simulink model "fir_ssr"  (R2023a)
settings: Solver=VariableStepAuto  StartTime=0.0  StopTime=5000  RelTol=1e-3
PreLoadFcn:
  | xmcCheckSlxPath(bdroot)
  | SSR4_init
InitFcn:
  | xmcCheckSlxPath(bdroot)
  | SSR4_init;
undefined symbols (not defined in the file): N, None, S, SHIFT_ACC, Taps, vsva2197, xcvc1902
libraries: aieBasic x8, aieUtilities x4, dspsrcs4 x1, simulink x1, vmcUtilities x1, aieDSP x1
settings Model: Creator=oliviert  LastModifiedBy=robg
settings SolverCC: AlgebraicLoopSolver=TrustRegion
settings DebuggingCC: UnconnectedInputMsg=warning  UnconnectedOutputMsg=warning  UnconnectedLineMsg=warning
settings ModelReferenceCC: EnableRefExpFcnMdlSchedulingChecks=on
settings RTWCC: DLArmComputeVersion=19.05

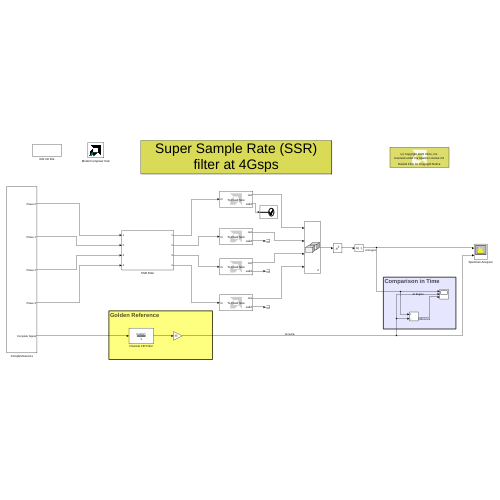
[thumbnail: Simulink's stored preview of the top-level diagram]
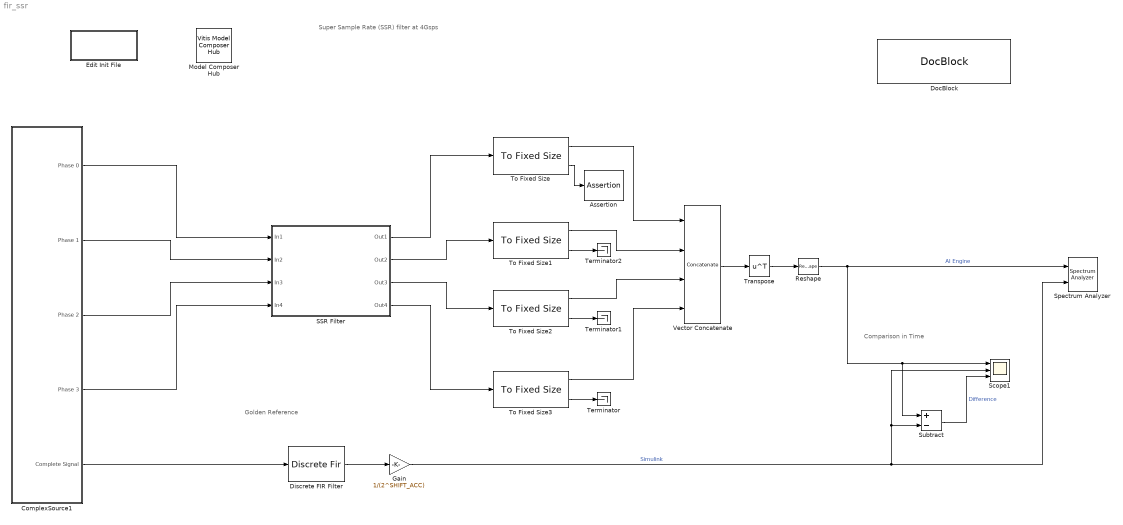
== system fir_ssr ==
  note: Comparison in Time
  note: Golden Reference
  note: Super Sample Rate (SSR) filter at 4Gsps
  Assertion : Assertion
  ComplexSource1 : Subsystem  mask{s=0}
      mask prompts: s "Seed"
  Discrete FIR Filter : DiscreteFir  Coefficients=Taps  InputProcessing=Columns as channels (frame based)
  DocBlock : simulink/Model-Wide Utilities/DocBlock  DocumentType=Text  mask(DocBlock){}
      content=|
      | ///////////////////////////////////////////////////////////////////////////
      | // Copyright 2020 Xilinx
      | //
      | // Licensed under the Apache License, Version 2.0 (the "License");
      | // you may not use this file except in compliance with the License.
      | // You may obtain a copy of the License at
      | //
      | // http://www.apache.org/licenses/LICENSE-2.0
      | //
      | // Unless required by applicable law or agreed to in writing, software
      | // distributed under the License is distributed on an "AS IS" BASIS,
      | // WITHOUT WARRANTIES OR CONDITIONS OF ANY KIND, either express or implied.
      | // See the License for the specific language governing permissions and
      | // limitations under the License.
      | ///////////////////////////////////////////////////////////////////////////
      mask Display:
      | xmcDrawBlockIcon();
      | disp(['{\fontsize{10pt}(c) Copyright 2022' ' Xilinx, Inc.}\newline \newline '],'texmode','on');
      | disp('{\fontsize{10pt}Licensed under the Apache License 2.0}','texmode','on');
      | disp('\newline \newline \newline{\fontsize{10pt}Double Click for Copyright Notice}','texmode','on');
  Edit Init File : Subsystem
      settings: OpenFcn=edit('SSR4_init.m');
  Gain : Gain  Gain=1/(2^SHIFT_ACC)
  Model Composer Hub : vmcUtilities/Vitis Model Composer Hub  Tag=genX  CodeGeneration=off  SubsystemName=SSR Filter  StartColumn=1  NumberOfColumns=1  TargetDirectory=./code_SSR4  exportDesign=off  analyzeDesign=off  validateDesignOnHw=off  ExportType=AI Engines  IpVendor=xilinx.com  IpLibrary=hls  IpVersion=1.0  IpHWLanguage=Verilog  AieCompilerOptions={}  AieSimulatorOptions={}  CreateTestbench=on  TestbenchStackSize=10  RunRtlSim=off  RunCSim=off  RunAieSim=on  AieSimTimeout=50000  RunAieSimProfiling=off  LaunchVitisAnalyzer=off  PlotOutput=on  RunX86Sim=off  X86SimTimeout=10  GenHwImage=off  GenLibadfXo=off  GenHwValidationCode=off  PlatformType=Not Specified  HwSystemType=Baremetal  HwValidationTarget=hw  ProjDevice=xcvc1902-vsva2197-1LP-e-S  ProjDevicePart=xcvc1902-vsva2197-1LP-e-S  AIEType=AIE  SamplePeriod=-1  ClockFrequency=200  DataPathParallelism=1  xilinxfamily=versalaicore  part=xcvc1902  speed=-2MP-e-S  package=vsva2197  directory=./netlist  testbench=off  incr_netlist=off  synthesis_tool=Vivado  clock_wrapper=Clock Enables  dbl_ovrd=According to Block Masks  dcm_input_clock_period=10  sysclk_period=10  simulink_period=1  eval_field=0  LogFileName=''  NThreads=4
  Reshape : Reshape
  SSR Filter : Subsystem
  Scope1 : Scope  NumInputPorts=3
  Spectrum Analyzer : SpectrumAnalyzer  NumInputPorts=2  WindowPosition=[1534 429 422 270]  Visible=on  Method=Welch  SampleRate=8  Span=8  StartFrequency=-4  StopFrequency=4  AveragingMethod=Exponential  YLimits=[-44.0464,106.8068]  ShowLegend=on  ChannelNames="[\"\"]"  DefaultConfigurationName=spbscopes.SpectrumAnalyzerBlockCfg
  Subtract : Sum  Inputs=+-
  Terminator : Terminator
  Terminator1 : Terminator
  Terminator2 : Terminator
  To Fixed Size{,1..3} (4 alike) : aieUtilities/To Fixed Size  Mode=Produce a valid output signal  OutputSize=Inherit: Same as input  CopyMethod=Buffer samples to form output  HasStatusOutput=off
  Transpose : Math  Operator=transpose
  Vector Concatenate : Concatenate  NumInputs=4  Mode=Multidimensional array  ConcatenateDimension=2
  wires:
  SSR Filter/2(Out2) -> To Fixed Size1/1
  To Fixed Size1/1 -> Vector Concatenate/2
  Reshape/1 -> Spectrum Analyzer/1, Subtract/1, Scope1/1  "AI Engine"
  SSR Filter/1(Out1) -> To Fixed Size/1
  Subtract/1 -> Scope1/3  "Difference"
  Vector Concatenate/1 -> Transpose/1
  To Fixed Size3/1 -> Vector Concatenate/4
  To Fixed Size2/1 -> Vector Concatenate/3
  Transpose/1 -> Reshape/1
  To Fixed Size/1 -> Vector Concatenate/1
  Discrete FIR Filter/1 -> Gain/1
  SSR Filter/3(Out3) -> To Fixed Size2/1
  Gain/1 -> Spectrum Analyzer/2, Subtract/2, Scope1/2  "Simulink"
  SSR Filter/4(Out4) -> To Fixed Size3/1
  ComplexSource1/3(Phase 2) -> SSR Filter/3(In3)
  ComplexSource1/4(Phase 3) -> SSR Filter/4(In4)
  ComplexSource1/1(Phase 0) -> SSR Filter/1(In1)
  ComplexSource1/2(Phase 1) -> SSR Filter/2(In2)
  ComplexSource1/5(Complete Signal) -> Discrete FIR Filter/1
  To Fixed Size/2 -> Assertion/1
  To Fixed Size3/2 -> Terminator/1
  To Fixed Size2/2 -> Terminator1/1
  To Fixed Size1/2 -> Terminator2/1

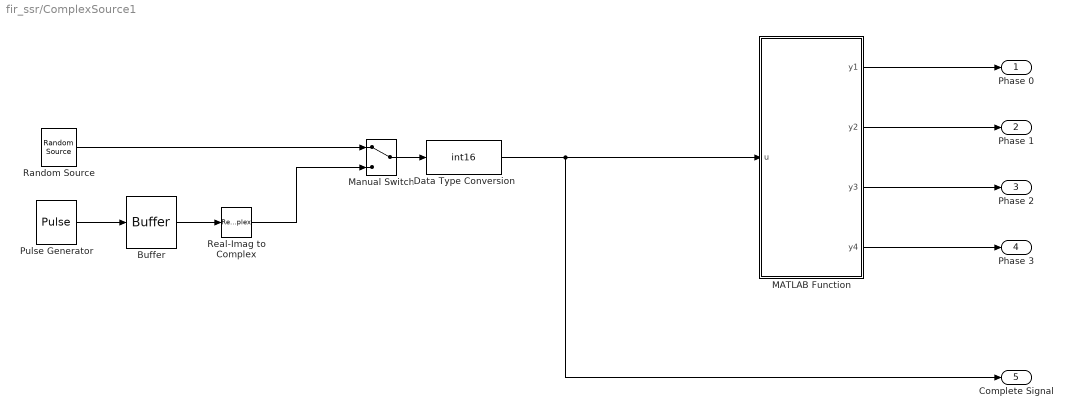
== system fir_ssr/ComplexSource1 ==
  Buffer : Buffer  N=N*4  OutputFrames=off
  Data Type Conversion : DataTypeConversion  OutDataTypeStr=int16  SaturateOnIntegerOverflow=off  RndMeth=Floor
  MATLAB Function : MATLAB Function  TreatAsAtomicUnit=on
  Manual Switch : ManualSwitch
  Pulse Generator : DiscretePulseGenerator  Amplitude=20000  Period=32 + 40*5  PhaseDelay=32  SampleTime=1/8
  Random Source : dspsrcs4/Random Source  SrcType=Uniform  NormMethod=Ziggurat  CltLength=12  MinVal=-20000  MaxVal=20000  MeanVal=0  VarVal=1  RepMode=Specify seed  rawSeed=s  IsInherit=off  SampMode=Discrete  SampTime=1/8  SampFrame=4*N  DataType=Double  OutComplex=Complex  OutputFrames=off
  Real-Imag to Complex : RealImagToComplex  Input=Real
  Phase 0 : Outport
  Phase 1 : Outport  Port=2
  Phase 2 : Outport  Port=3
  Phase 3 : Outport  Port=4
  Complete Signal : Outport  Port=5
  wires:
  MATLAB Function/1(y1) -> Phase 0/1
  MATLAB Function/2(y2) -> Phase 1/1
  MATLAB Function/3(y3) -> Phase 2/1
  MATLAB Function/4(y4) -> Phase 3/1
  Real-Imag to Complex/1 -> Manual Switch/2
  Pulse Generator/1 -> Buffer/1
  Data Type Conversion/1 -> Complete Signal/1, MATLAB Function/1(u)
  Buffer/1 -> Real-Imag to Complex/1
  Manual Switch/1 -> Data Type Conversion/1
  Random Source/1 -> Manual Switch/1

== system fir_ssr/Edit Init File ==

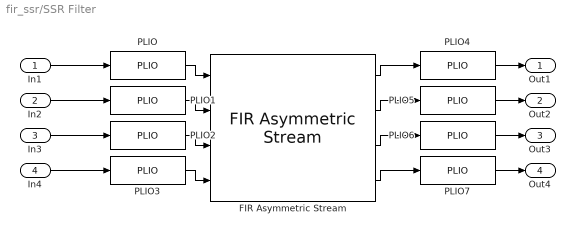
== system fir_ssr/SSR Filter ==
  In1 : Inport
  In2 : Inport  Port=2
  In3 : Inport  Port=3
  In4 : Inport  Port=4
  FIR Asymmetric Stream : aieDSP/FIR Asymmetric Stream  data_type=cint16  coef_type=cint16  use_coeff_reload=off  dual_ip=off  num_outputs=off  coeff=Taps  fir_length=28  input_window_size=N*4  shift_val=SHIFT_ACC  rnd_mode=Round to positive infinity  sat_mode=0-None  ssr=NPHASES  casc_length=1  AIE_VARIANT=1  blockJsonConstraints=[]  blockJsonConstraintsInternal=[]  spec=vmc_stream_fir_sr_asym.json  SerializedMaskParamNames=[]  SerializedMaskParamValues=[]  SerializedMaskParamVisibilities=[]  block_type=FIR Asymmetric Stream  SerializedMaskParamDataypes=typename|typename|bool|bool|bool|coef_type|uint|uint|uint|uint|uint|uint|uint|uint  SerializedMaskParamEnumStrArr=0|0|0|0|0|0|0|0|0|Floor,Ceiling,Round to positive infinity,Round to negative infinity,Round symmetrical to infinity,Round symmetrical to zero,Round convergent to even,Round convergent to odd|0-None,1-Asymmetric,3-Symmetric|0|0|0  SerializedMaskParamEnumValArr=0|0|0|0|0|0|0|0|0|0,1,2,3,4,5,6,7|0,1,3|0|0|0  SerializedMaskParamVectorArr=0|0|0|0|0|1|0|0|0|0|0|0|0|0
  PLIO{,1..7} (8 alike) : aieBasic/PLIO  PlioWidth=64  PlioFreqSpec=on  PlioFreq=PLIO_FREQ  ColLocation=0  channel=0  blockJsonConstraints=[]  deprecateConstraints=0
  Out1 : Outport
  Out2 : Outport  Port=2
  Out3 : Outport  Port=3
  Out4 : Outport  Port=4
  wires:
  In4/1 -> PLIO3/1
  In1/1 -> PLIO/1
  FIR Asymmetric Stream/4 -> PLIO7/1
  FIR Asymmetric Stream/1 -> PLIO4/1
  In2/1 -> PLIO1/1
  In3/1 -> PLIO2/1
  FIR Asymmetric Stream/2 -> PLIO5/1
  FIR Asymmetric Stream/3 -> PLIO6/1
  PLIO/1 -> FIR Asymmetric Stream/1
  PLIO1/1 -> FIR Asymmetric Stream/2
  PLIO2/1 -> FIR Asymmetric Stream/3
  PLIO3/1 -> FIR Asymmetric Stream/4
  PLIO4/1 -> Out1/1
  PLIO5/1 -> Out2/1
  PLIO6/1 -> Out3/1
  PLIO7/1 -> Out4/1

== matlab function fir_ssr/ComplexSource1/MATLAB Function ==
  data: u input; y1 output; y2 output; y3 output; y4 output
function [y1,y2,y3,y4] = fcn(u)

y1 = u(1:4:end);
y2 = u(2:4:end);
y3 = u(3:4:end);
y4 = u(4:4:end);
